simulink model "Simulink_StateDerivVec"  (R2022a)
settings: Solver=FixedStepAuto  StartTime=0.0  StopTime=timeEnd  FixedStep=SampleTime  RelTol=1e-6
values from neighbouring files (symbols this model uses):
  HorDistData = HorDistVec    [MainScript.m]    (also in MainScript_function.m)
  HorForceData = HorForceVec    [MainScript.m]    (also in MainScript_function.m)
  InitAIFactorVec = 1/3*ones(Farm.NumTurb,1)    [MainScript.m]    (also in MainScript_function.m)
  InitBladePitch = 0*ones(Farm.NumTurb,1)    [MainScript.m]    (also in MainScript_function.m)
  InitFreeStreamWindVel = Global.MeanWindSpeed    [MainScript.m]    (also in MainScript_function.m)
  InitGeneTorqueVec = 30000.*ones(Farm.NumTurb,1) * 97    [MainScript.m]    (also in MainScript_function.m)
  InitRotorSpeedVec = 1*ones(Farm.NumTurb,1)    [MainScript.m]    (also in MainScript_function.m)
  InitStateVec = [ ... (first row only)    [MainScript.m]    (also in MainScript_function.m)
  InitYawAngleVec = [-15;15;0]*pi/180    [MainScript.m]    (also in MainScript_function.m)
  modelselect = 1    [MainScript.m]    (also in MainScript_function.m)
  SampleTime = 1    [MainScript.m]    (also in MainScript_function.m)
settings Model: Creator=alich  LastModifiedBy=mluser
settings SolverCC: AlgebraicLoopSolver=LineSearch
settings DataIOCC: ExternalInput=Moor
settings DebuggingCC: UnconnectedInputMsg=warning  UnconnectedOutputMsg=warning  UnconnectedLineMsg=warning  SFMachineParentedDataDiag=warning
settings SFSimCC: CustomCodeUndefinedFunction=UseInterfaceOnly  DefaultCustomCodeDeterministicFunctions=All
settings RTWCC: GenCodeOnly=on  DLArmComputeVersion=19.05

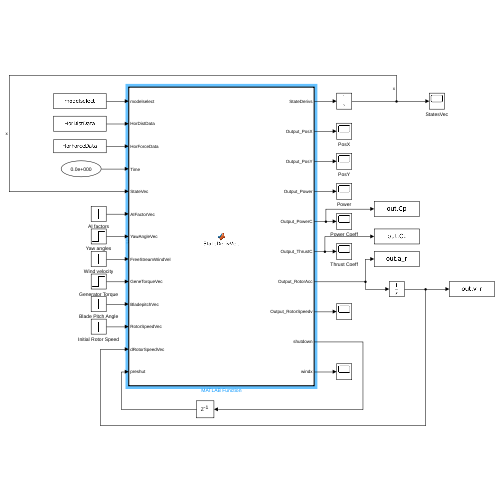
[thumbnail: Simulink's stored preview of the top-level diagram]
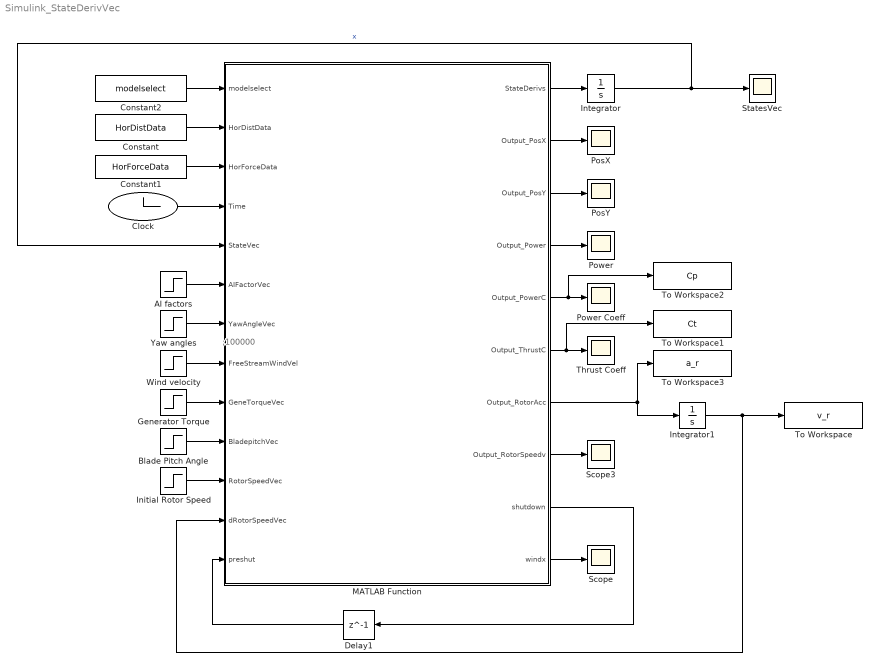
== system Simulink_StateDerivVec ==
  note: ;100000
  AI factors : Step  Time=0  Before=InitAIFactorVec  After=InitAIFactorVec  SampleTime=SampleTime
  Blade Pitch Angle : Step  Time=0  Before=InitBladePitch  After=InitBladePitch  SampleTime=SampleTime
  Clock : Clock
  Constant : Constant  Value=HorDistData  VectorParams1D=off
  Constant1 : Constant  Value=HorForceData  VectorParams1D=off
  Constant2 : Constant  Value=modelselect  SampleTime=SampleTime
  Delay1 : Delay  DelayLength=1  InitialCondition=0  SampleTime=SampleTime
  Generator Torque : Step  Time=0  Before=InitGeneTorqueVec  After=InitGeneTorqueVec  SampleTime=SampleTime
  Initial Rotor Speed : Step  Time=0  Before=InitRotorSpeedVec  After=InitRotorSpeedVec  SampleTime=SampleTime
  Integrator : Integrator  InitialCondition=InitStateVec  UpperSaturationLimit=100000  LowerSaturationLimit=0  IgnoreLimit=on
  Integrator1 : Integrator
  MATLAB Function : MATLAB Function  TreatAsAtomicUnit=on
  PosX : Scope
  PosY : Scope
  Power : Scope
  Power Coeff : Scope
  Scope : Scope
  Scope3 : Scope
  StatesVec : Scope
  Thrust Coeff : Scope
  To Workspace : ToWorkspace  VariableName=v_r  SaveFormat=Timeseries  SampleTime=-1
  To Workspace1 : ToWorkspace  VariableName=Ct  SaveFormat=Timeseries  SampleTime=-1
  To Workspace2 : ToWorkspace  VariableName=Cp  SaveFormat=Timeseries  SampleTime=-1
  To Workspace3 : ToWorkspace  VariableName=a_r  SaveFormat=Timeseries  SampleTime=-1
  Wind velocity : Step  Time=0  Before=[InitFreeStreamWindVel,0]  After=[InitFreeStreamWindVel,0]  SampleTime=SampleTime
  Yaw angles : Step  Time=0  Before=InitYawAngleVec  After=InitYawAngleVec  SampleTime=SampleTime
  wires:
  Clock/1 -> MATLAB Function/4(Time)
  MATLAB Function/1(StateDerivs) -> Integrator/1
  Integrator/1 -> MATLAB Function/5(StateVec), StatesVec/1  "x"
  MATLAB Function/2(Output_PosX) -> PosX/1
  MATLAB Function/3(Output_PosY) -> PosY/1
  MATLAB Function/4(Output_Power) -> Power/1
  AI factors/1 -> MATLAB Function/6(AIFactorVec)
  Yaw angles/1 -> MATLAB Function/7(YawAngleVec)
  Wind velocity/1 -> MATLAB Function/8(FreeStreamWindVel)
  MATLAB Function/5(Output_PowerC) -> Power Coeff/1, To Workspace2/1
  MATLAB Function/7(Output_RotorAcc) -> To Workspace3/1, Integrator1/1
  Initial Rotor Speed/1 -> MATLAB Function/11(RotorSpeedVec)
  Generator Torque/1 -> MATLAB Function/9(GeneTorqueVec)
  Integrator1/1 -> MATLAB Function/12(dRotorSpeedVec), To Workspace/1
  MATLAB Function/6(Output_ThrustC) -> Thrust Coeff/1, To Workspace1/1
  Blade Pitch Angle/1 -> MATLAB Function/10(BladepitchVec)
  MATLAB Function/8(Output_RotorSpeedv) -> Scope3/1
  MATLAB Function/9(shutdown) -> Delay1/1
  Delay1/1 -> MATLAB Function/13(preshut)
  MATLAB Function/10(windx) -> Scope/1
  Constant/1 -> MATLAB Function/2(HorDistData)
  Constant1/1 -> MATLAB Function/3(HorForceData)
  Constant2/1 -> MATLAB Function/1(modelselect)

== matlab function Simulink_StateDerivVec/MATLAB Function ==
  data: modelselect input; HorDistData input; HorForceData input; Time input; StateDerivs output; StateVec input; AIFactorVec input; YawAngleVec input; FreeStreamWindVel input; GeneTorqueVec input; BladepitchVec input; Output_PosX output; Output_PosY output; Output_Power output; Output_PowerC output; Output_ThrustC output; RotorSpeedVec input; Output_RotorAcc output; dRotorSpeedVec input; Output_RotorSpeedv output; preshut input; shutdown output; windx output
function [StateDerivs,Output_PosX,Output_PosY,Output_Power,Output_PowerC,Output_ThrustC,Output_RotorAcc,Output_RotorSpeedv,shutdown,windx]    = StateDerivVec(modelselect,HorDistData,HorForceData,Time,StateVec,AIFactorVec,YawAngleVec,FreeStreamWindVel,GeneTorqueVec,BladepitchVec,RotorSpeedVec,dRotorSpeedVec,preshut)
%% Load structures

Pars = load('Parameters_Simu.mat');

Solver = Pars.Solver; 
Global = Pars.Global;
Farm = Pars.Farm;
Turb = Pars.Turb;
Moor = Pars.Moor;
Arrays = Pars.Arrays;
TurbPosStateDerivMat = Arrays.TurbPosStateDerivMat;
TurbVelStateDerivMat = Arrays.TurbVelStateDerivMat;
WakeStateDerivMat = Arrays.WakeStateDerivMat;
TurbPowerVec = Arrays.TurbPowerVec;
WakeLocalVel = Arrays.WakeLocalVel;
WakeLocalAccel = Arrays.WakeLocalAccel;
WakeLocalDiaROT = Arrays.WakeLocalDiaROT;
Output_PosX = Arrays.Output_PosX;
Output_PosY = Arrays.Output_PosY;
Output_Power = Arrays.Output_Power;
Output_ThrustC=Arrays.Output_Power;
Output_PowerC=Arrays.Output_Power;
Output_RotorAcc=Arrays.Output_Power;
Output_RotorSpeedv = Arrays.Output_Power;
shutdown = Arrays.Output_Power;
windx = Arrays.Output_Power;

%if(modelselect==1)
data=load('paraVal.mat');
Lambda.mesh=data.paraVal.aero.lambda_grid;
Beta.mesh=data.paraVal.aero.beta_grid;
Cp.mesh=data.paraVal.aero.cp_grid;
Ct.mesh=data.paraVal.aero.ct_grid;
%end
   
%% Extract states and inputs
TurbPosMat = reshape(StateVec(1:2*Farm.NumTurb),2,Farm.NumTurb);
TurbVelMat = reshape(StateVec(2*Farm.NumTurb + 1:4*Farm.NumTurb),2,Farm.NumTurb);
WakeStateMat = reshape(StateVec(4*Farm.NumTurb + 1:4*Farm.NumTurb + 4*Farm.TotalNumWakePoints),4,Farm.TotalNumWakePoints);
for TurbNum = 1:Farm.NumTurb
 % Turbine states
 Turb(TurbNum).PosVec = TurbPosMat(:,TurbNum);
 Turb(TurbNum).VelVec = TurbVelMat(:,TurbNum);
 
 % Wake states
 Turb(TurbNum).WakePointPos_Y(1:Turb(TurbNum).NumWakePoints) = WakeStateMat(1,1:Turb(TurbNum).NumWakePoints);
 Turb(TurbNum).WakePointVelVec(:,1:Turb(TurbNum).NumWakePoints) = WakeStateMat(2:3,1:Turb(TurbNum).NumWakePoints);
 Turb(TurbNum).WakePointDia(1:Turb(TurbNum).NumWakePoints) = WakeStateMat(4,1:Turb(TurbNum).NumWakePoints);
 WakeStateMat(:,1:Turb(TurbNum).NumWakePoints) = [];
 
 % Turbine inputs
 Turb(TurbNum).YawAngle = YawAngleVec(TurbNum); %Yaw angle input is the same for both version of the model
 
 if(modelselect ==1) %3input
 Turb(TurbNum).BladePitch=BladepitchVec(TurbNum);
 Turb(TurbNum).GeneTorque=GeneTorqueVec(TurbNum);

 if (Time==0)
     Turb(TurbNum).RotorSpeed=RotorSpeedVec(TurbNum);
 else
     Turb(TurbNum).RotorSpeed=RotorSpeedVec(TurbNum)+dRotorSpeedVec(TurbNum);
     
 end
 else
     Turb(TurbNum).AIFactor = AIFactorVec(TurbNum);
 end
 
 end
 
% Free stream wind condition
Global.FreeStreamWindVel = FreeStreamWindVel; 
Global.FreeStreamWindAccel = [0 0]';

%% Define free stream wind unit vector
Global.FreeStreamUnitVec = Global.FreeStreamWindVel/norm(Global.FreeStreamWindVel);

%% Begin loop for state derivatives
BaseNum = 0;
for TurbNum = 1:Farm.NumTurb

 %% Calculate turbine platform state-derivatives
 % Incident wind velocity
 if (TurbNum == 1)
  Turb(TurbNum).UpsWindVelVec = Global.FreeStreamWindVel;
 else
  EffVelDeficit = 0;
  for UpsTurbNum = 1:TurbNum - 1
      if(preshut(TurbNum-1)==1&& UpsTurbNum>1)
     UpsTurbNum1 = UpsTurbNum-1;%check
      else
          UpsTurbNum1 = UpsTurbNum;
      end
      
   TurbPosXRelUpsTurb = Turb(TurbNum).PosVec(1) - Turb(UpsTurbNum1).PosVec(1);
   if TurbPosXRelUpsTurb >= 0
    UpsWakePosXData = [0 Turb(UpsTurbNum1).WakePointPos_X(1:Turb(TurbNum).NumWakePoints)];
    UpsWakePosYData = [0 Turb(UpsTurbNum1).WakePointPos_Y(1:Turb(TurbNum).NumWakePoints)];
    UpsWakeVelXData = [Turb(UpsTurbNum1).InitWakeVelVec(1) Turb(UpsTurbNum1).WakePointVelVec(1,1:Turb(TurbNum).NumWakePoints)];
    UpsWakeVelYData = [Turb(UpsTurbNum1).InitWakeVelVec(2) Turb(UpsTurbNum1).WakePointVelVec(2,1:Turb(TurbNum).NumWakePoints)];
    UpsWakeDiaData = [Turb(UpsTurbNum1).RotorDia Turb(UpsTurbNum1).WakePointDia(1:Turb(TurbNum).NumWakePoints)];
    
    for index = 1:length(UpsWakeVelXData) %in case of special numerical issue.
    if(isnan(UpsWakeVelXData(index))||isinf(UpsWakeVelXData(index)))
        UpsWakeVelXData(index) = 0;
    end
    end
    
    for indexs = 1:length(UpsWakeVelYData)
    if(isnan(UpsWakeVelYData(indexs))||isinf(UpsWakeVelYData(indexs)))
        UpsWakeVelYData(indexs) = 0;
    end
    end
    
    
    UpsWakePosY = Turb(UpsTurbNum1).PosVec(2) + interp1(UpsWakePosXData,UpsWakePosYData,TurbPosXRelUpsTurb,'Spline');
    UpsWakeVelX = Turb(UpsTurbNum1).VelVec(1) + interp1(UpsWakePosXData,UpsWakeVelXData,TurbPosXRelUpsTurb,'Spline');
    UpsWakeVelY = Turb(UpsTurbNum1).VelVec(2) + interp1(UpsWakePosXData,UpsWakeVelYData,TurbPosXRelUpsTurb,'Spline');
    UpsWakeDia = interp1(UpsWakePosXData,UpsWakeDiaData,TurbPosXRelUpsTurb,'Spline');
    UpsWakeOffset = abs(UpsWakePosY - Turb(TurbNum).PosVec(2));
    if UpsWakeOffset >= Turb(TurbNum).RotorDia/2 + UpsWakeDia/2
     EffVelVec = Global.FreeStreamWindVel;
    else
     b = Turb(TurbNum).RotorDia*(Global.GaussStd_Slope*TurbPosXRelUpsTurb/Turb(TurbNum).RotorDia + Global.GaussStd_Inter);
     a_x = 0.5*(((UpsWakeDia/2)/b)^2)*([1 0]*Global.FreeStreamWindVel - UpsWakeVelX);
     a_y = 0.5*(((UpsWakeDia/2)/b)^2)*([0 1]*Global.FreeStreamWindVel - UpsWakeVelY);
     UpsWakeVelX_Gauss = @(r) [1 0]*Global.FreeStreamWindVel - a_x*exp(-(r.^2)/(2*(b^2)));
     UpsWakeVelY_Gauss = @(r) [0 1]*Global.FreeStreamWindVel - a_y*exp(-(r.^2)/(2*(b^2)));
     Func_x = @(r) r.*AngleOLFunc(UpsWakeOffset,r,Turb(TurbNum).RotorDia/2).*UpsWakeVelX_Gauss(r);
     Func_y = @(r) r.*AngleOLFunc(UpsWakeOffset,r,Turb(TurbNum).RotorDia/2).*UpsWakeVelY_Gauss(r);
     r_vec = linspace(max(UpsWakeOffset - Turb(UpsTurbNum1).RotorDia/2,0),UpsWakeOffset + Turb(TurbNum).RotorDia/2,10);
     EffVelVec = [
      trapz(r_vec,Func_x(r_vec))/Turb(TurbNum).RotorArea;
      trapz(r_vec,Func_y(r_vec))/Turb(TurbNum).RotorArea];
     
    end
    EffVelDeficit =...
     EffVelDeficit + (norm(Global.FreeStreamWindVel)...
     - dot(EffVelVec,Global.FreeStreamUnitVec))^2;
   end
  end
  Turb(TurbNum).UpsWindVelVec =...
   (norm(Global.FreeStreamWindVel)...
   - sqrt(EffVelDeficit))*Global.FreeStreamUnitVec;

if(Turb(TurbNum).UpsWindVelVec(1)<0)
    Turb(TurbNum).UpsWindVelVec(1) = 0;
end
if(Turb(TurbNum).UpsWindVelVec(2)<0)
    Turb(TurbNum).UpsWindVelVec(2) = 0;
end


    
 end

 
 %% Ali's model to find Power and Thrust coefficients
 % Aerodynamic thrust force
 Turb(TurbNum).RelUpsWindVelVec = Turb(TurbNum).UpsWindVelVec - Turb(TurbNum).VelVec;
 Turb(TurbNum).RelWindAngle = atan(Turb(TurbNum).RelUpsWindVelVec(2)/Turb(TurbNum).RelUpsWindVelVec(1));
 Turb(TurbNum).RelYawAngle = Turb(TurbNum).YawAngle - Turb(TurbNum).RelWindAngle; %

 if(modelselect == 1)
 Turb(TurbNum).NormalWindVel = norm(Turb(TurbNum).RelUpsWindVelVec)*cos(Turb(TurbNum).RelYawAngle);%82
 Turb(TurbNum).Lambda = Turb(TurbNum).RotorSpeed*Turb(TurbNum).RotorDia/2/Turb(TurbNum).NormalWindVel;

 Turb(TurbNum).PowerCoeff = interp2(Beta.mesh,Lambda.mesh,Cp.mesh,Turb(TurbNum).BladePitch,Turb(TurbNum).Lambda);
 Turb(TurbNum).ThrustCoeff = interp2(Beta.mesh,Lambda.mesh,Ct.mesh,Turb(TurbNum).BladePitch,Turb(TurbNum).Lambda); 

 Turb(TurbNum).TurbTorque = 0.5*Global.AirDensity*Turb(TurbNum).RotorArea*(Turb(TurbNum).NormalWindVel)^3*Turb(TurbNum).PowerCoeff/Turb(TurbNum).RotorSpeed;
 Output_RotorAcc(TurbNum) = (Turb(TurbNum).TurbTorque-Turb(TurbNum).GeneTorque)/Turb(TurbNum).MomentInertia;

 if(isinf( Output_RotorAcc(TurbNum))||isnan( Output_RotorAcc(TurbNum)))
      Output_RotorAcc(TurbNum)=0;
      
 end
 else
    if(Turb(TurbNum).UpsWindVelVec(1)<=3) %%check
      Turb(TurbNum).AIFactor = 0;
    else
     Turb(TurbNum).AIFactor = AIFactorVec(TurbNum);
    end
  if strcmp(Solver.ActDiscModel,'Momentum')
  Turb(TurbNum).ThrustCoeff = 4*Turb(TurbNum).AIFactor*(cos(Turb(TurbNum).RelYawAngle) - Turb(TurbNum).AIFactor);
  Turb(TurbNum).PowerCoeff = 4*Turb(TurbNum).AIFactor*((cos(Turb(TurbNum).RelYawAngle) - Turb(TurbNum).AIFactor)^2); %fsolve
 elseif strcmp(Solver.ActDiscModel,'Glauert')
  Turb(TurbNum).ThrustCoeff = 4*Turb(TurbNum).AIFactor*sqrt(1 - Turb(TurbNum).AIFactor*(2*cos(Turb(TurbNum).RelYawAngle) - Turb(TurbNum).AIFactor));
  Turb(TurbNum).PowerCoeff = 4*Turb(TurbNum).AIFactor*(cos(Turb(TurbNum).RelYawAngle) - Turb(TurbNum).AIFactor)*sqrt(1 - Turb(TurbNum).AIFactor*(2*cos(Turb(TurbNum).RelYawAngle) - Turb(TurbNum).AIFactor));
 elseif strcmp(Solver.ActDiscModel,'Vortex')
  DefAngle = (0.6*Turb(TurbNum).AIFactor + 1)*Turb(TurbNum).RelYawAngle;
  Turb(TurbNum).ThrustCoeff = 4*Turb(TurbNum).AIFactor*(cos(Turb(TurbNum).RelYawAngle) + tan(DefAngle/2)*sin(Turb(TurbNum).RelYawAngle) - Turb(TurbNum).AIFactor*((sec(DefAngle/2))^2));
  Turb(TurbNum).PowerCoeff = 4*Turb(TurbNum).AIFactor*(cos(Turb(TurbNum).RelYawAngle) - Turb(TurbNum).AIFactor)*(cos(Turb(TurbNum).RelYawAngle) + tan(DefAngle/2)*sin(Turb(TurbNum).RelYawAngle) - Turb(TurbNum).AIFactor*((sec(DefAngle/2))^2));
 else
  error('Selected actuator disc model does not exist...');
  end
 end
     
 Turb(TurbNum).RotorNormVec = [
  cos(Turb(TurbNum).YawAngle);
  sin(Turb(TurbNum).YawAngle)];
 Turb(TurbNum).ThrustForceVec =...
  0.5*Turb(TurbNum).ThrustCoeff*Global.AirDensity*Turb(TurbNum).RotorArea*...
  (norm(Turb(TurbNum).RelUpsWindVelVec)^2)*Turb(TurbNum).RotorNormVec;
 
 
 % Hydrodynamic drag force
 Turb(TurbNum).DragForceVec = -Turb(TurbNum).EffDragFactor*norm(Turb(TurbNum).VelVec)*Turb(TurbNum).VelVec;
 LinDampForceVec = -1000000*Turb(TurbNum).VelVec;
 
 % Mooring line restoring force
 FLPosRelAnch1 = Turb(TurbNum).PosVec + Turb(TurbNum).FL1PosRelG - Turb(TurbNum).Anch1PosVec;
 FLPosRelAnch2 = Turb(TurbNum).PosVec + Turb(TurbNum).FL2PosRelG - Turb(TurbNum).Anch2PosVec;
 FLPosRelAnch3 = Turb(TurbNum).PosVec + Turb(TurbNum).FL3PosRelG - Turb(TurbNum).Anch3PosVec;
 Line1HorDist = norm(FLPosRelAnch1);
 Line2HorDist = norm(FLPosRelAnch2);
 Line3HorDist = norm(FLPosRelAnch3);
 Line1HorForce = interp1(HorDistData,HorForceData,Line1HorDist,'Spline');
 Line2HorForce = interp1(HorDistData,HorForceData,Line2HorDist,'Spline');
 Line3HorForce = interp1(HorDistData,HorForceData,Line3HorDist,'Spline');
 MoorForce1 = -Line1HorForce*FLPosRelAnch1/Line1HorDist;
 MoorForce2 = -Line2HorForce*FLPosRelAnch2/Line2HorDist;
 MoorForce3 = -Line3HorForce*FLPosRelAnch3/Line3HorDist;
 Turb(TurbNum).MoorForceVec = MoorForce1 + MoorForce2 + MoorForce3;
 
 % Turbine acceleration
 Turb(TurbNum).ForceVec = Turb(TurbNum).ThrustForceVec + Turb(TurbNum).MoorForceVec + Turb(TurbNum).DragForceVec...
     + LinDampForceVec;
 Turb(TurbNum).AccelVec = Solver.TurbMotion*Turb(TurbNum).ForceVec/(Turb(TurbNum).Mass + Turb(TurbNum).AddedMass);
 
 % Turbine power calculation
 
 if(modelselect ==1)
  if(preshut(TurbNum)==0)
 Turb(TurbNum).Power = Turb(TurbNum).RotorSpeed*Turb(TurbNum).GeneTorque;
 
 
 TurbPowerVec(TurbNum) = Turb(TurbNum).Power;
  else
  TurbPowerVec(TurbNum) = 0;
  end
 else
     Turb(TurbNum).Power = 0.5*Turb(TurbNum).PowerCoeff*Global.AirDensity*Turb(TurbNum).RotorArea*(norm(Turb(TurbNum).RelUpsWindVelVec)^3) + 5*(TurbPosMat(1, TurbNum) - Turb(TurbNum).PosVec(1)) + 5*(TurbPosMat(2, TurbNum) - Turb(TurbNum).PosVec(2));
 TurbPowerVec(TurbNum) = Turb(TurbNum).Power;
 %% calculate power coeff with 5MW -> calculate AI
 Maxpower = 5/0.994; % maximum rated power is 5MW
 Turb(TurbNum).PowerCoeff = Maxpower/(0.5*Global.AirDensity*Turb(TurbNum).RotorArea*(norm(Turb(TurbNum).RelUpsWindVelVec)^3));
 if strcmp(Solver.ActDiscModel,'Momentum')
  Turb(TurbNum).PowerCoeff = 4*Turb(TurbNum).AIFactor*((cos(Turb(TurbNum).RelYawAngle) - Turb(TurbNum).AIFactor)^2); %fsolve
 elseif strcmp(Solver.ActDiscModel,'Glauert')
  Turb(TurbNum).ThrustCoeff = 4*Turb(TurbNum).AIFactor*sqrt(1 - Turb(TurbNum).AIFactor*(2*cos(Turb(TurbNum).RelYawAngle) - Turb(TurbNum).AIFactor));
  Turb(TurbNum).PowerCoeff = 4*Turb(TurbNum).AIFactor*(cos(Turb(TurbNum).RelYawAngle) - Turb(TurbNum).AIFactor)*sqrt(1 - Turb(TurbNum).AIFactor*(2*cos(Turb(TurbNum).RelYawAngle) - Turb(TurbNum).AIFactor));
 elseif strcmp(Solver.ActDiscModel,'Vortex')
  DefAngle = (0.6*Turb(TurbNum).AIFactor + 1)*Turb(TurbNum).RelYawAngle;
  Turb(TurbNum).ThrustCoeff = 4*Turb(TurbNum).AIFactor*(cos(Turb(TurbNum).RelYawAngle) + tan(DefAngle/2)*sin(Turb(TurbNum).RelYawAngle) - Turb(TurbNum).AIFactor*((sec(DefAngle/2))^2));
  Turb(TurbNum).PowerCoeff = 4*Turb(TurbNum).AIFactor*(cos(Turb(TurbNum).RelYawAngle) - Turb(TurbNum).AIFactor)*(cos(Turb(TurbNum).RelYawAngle) + tan(DefAngle/2)*sin(Turb(TurbNum).RelYawAngle) - Turb(TurbNum).AIFactor*((sec(DefAngle/2))^2));
 else
  error('Selected actuator disc model does not exist...');
 end
 end
  
 %% Calculate wake state derivatives
 % Boundary condition at turbine
 if strcmp(Solver.RotorMomModel,'Jimenez')
  InitWakeVelMag = norm(Turb(TurbNum).RelUpsWindVelVec)*sqrt(abs(1 - Turb(TurbNum).ThrustCoeff));
  InitWakeAngle = -((cos(Turb(TurbNum).RelYawAngle))^2)*sin(Turb(TurbNum).RelYawAngle)*Turb(TurbNum).ThrustCoeff/2;
  Turb(TurbNum).InitWakeVelVec = InitWakeVelMag*[
   cos(InitWakeAngle + Turb(TurbNum).RelWindAngle);
   sin(InitWakeAngle + Turb(TurbNum).RelWindAngle)];
 elseif strcmp(Solver.RotorMomModel,'Bastankhah')
  InitWakeVelMag = norm(Turb(TurbNum).RelUpsWindVelVec)*sqrt(1 - Turb(TurbNum).ThrustCoeff);
  InitWakeAngle = -0.3*Turb(TurbNum).RelYawAngle/cos(Turb(TurbNum).RelYawAngle)*(1 - sqrt(1 - Turb(TurbNum).ThrustCoeff*cos(Turb(TurbNum).RelYawAngle)));
  Turb(TurbNum).InitWakeVelVec = InitWakeVelMag*[
   cos(InitWakeAngle + Turb(TurbNum).RelWindAngle);
   sin(InitWakeAngle + Turb(TurbNum).RelWindAngle)];
 else
  error('Selected momentum model does not exist...');
 end

 
 % Wake propagation
 for PointNum = 1:Turb(TurbNum).NumWakePoints
  PropVel = [1 0]*Global.FreeStreamWindVel - Turb(TurbNum).VelVec(1);
  WakeRecovGrad = (1/(pi/4*Turb(TurbNum).WakePointDia(PointNum)^2))*(pi/2*Turb(TurbNum).WakePointDia(PointNum)*Global.WakeExpRate)*(Global.FreeStreamWindVel - (Turb(TurbNum).VelVec + Turb(TurbNum).WakePointVelVec(:,PointNum)));
  if PointNum == 1
   WakeLocalVel(PointNum) = Turb(TurbNum).WakePointVelVec(2,PointNum) - PropVel*(Turb(TurbNum).WakePointPos_Y(PointNum + Solver.CentralDiff))/Turb(TurbNum).WakePointPos_X(PointNum + Solver.CentralDiff);
   WakeLocalAccel(:,PointNum) = Global.FreeStreamWindAccel - Turb(TurbNum).AccelVec - PropVel*(Turb(TurbNum).WakePointVelVec(:,PointNum + Solver.CentralDiff) - Turb(TurbNum).InitWakeVelVec)/Turb(TurbNum).WakePointPos_X(PointNum + Solver.CentralDiff) + WakeRecovGrad;
   WakeLocalDiaROT(PointNum) = Global.WakeExpRate - PropVel*(Turb(TurbNum).WakePointDia(PointNum + Solver.CentralDiff) - Turb(TurbNum).RotorDia)/Turb(TurbNum).WakePointPos_X(PointNum + Solver.CentralDiff);
  elseif PointNum == Turb(TurbNum).NumWakePoints
   WakeLocalVel(PointNum) = Turb(TurbNum).WakePointVelVec(2,PointNum) - PropVel*(Turb(TurbNum).WakePointPos_Y(PointNum) - Turb(TurbNum).WakePointPos_Y(PointNum - 1))/(Turb(TurbNum).WakePointPos_X(PointNum) - Turb(TurbNum).WakePointPos_X(PointNum - 1));
   WakeLocalAccel(:,PointNum) = Global.FreeStreamWindAccel - Turb(TurbNum).AccelVec - PropVel*(Turb(TurbNum).WakePointVelVec(:,PointNum) - Turb(TurbNum).WakePointVelVec(:,PointNum - 1))/(Turb(TurbNum).WakePointPos_X(PointNum) - Turb(TurbNum).WakePointPos_X(PointNum - 1)) + WakeRecovGrad;
   WakeLocalDiaROT(PointNum) = Global.WakeExpRate - PropVel*(Turb(TurbNum).WakePointDia(PointNum) - Turb(TurbNum).WakePointDia(PointNum - 1))/(Turb(TurbNum).WakePointPos_X(PointNum) - Turb(TurbNum).WakePointPos_X(PointNum - 1));
  else
   WakeLocalVel(PointNum) = Turb(TurbNum).WakePointVelVec(2,PointNum) - PropVel*(Turb(TurbNum).WakePointPos_Y(PointNum + Solver.CentralDiff) - Turb(TurbNum).WakePointPos_Y(PointNum - 1))/(Turb(TurbNum).WakePointPos_X(PointNum + Solver.CentralDiff) - Turb(TurbNum).WakePointPos_X(PointNum - 1));
   WakeLocalAccel(:,PointNum) = Global.FreeStreamWindAccel - Turb(TurbNum).AccelVec - PropVel*(Turb(TurbNum).WakePointVelVec(:,PointNum + Solver.CentralDiff) - Turb(TurbNum).WakePointVelVec(:,PointNum - 1))/(Turb(TurbNum).WakePointPos_X(PointNum + Solver.CentralDiff) - Turb(TurbNum).WakePointPos_X(PointNum - 1)) + WakeRecovGrad;
   WakeLocalDiaROT(PointNum) = Global.WakeExpRate - PropVel*(Turb(TurbNum).WakePointDia(PointNum + Solver.CentralDiff) - Turb(TurbNum).WakePointDia(PointNum - 1))/(Turb(TurbNum).WakePointPos_X(PointNum + Solver.CentralDiff) - Turb(TurbNum).WakePointPos_X(PointNum - 1));
  end
 end 
 
 % Build state derivative matrices
 TurbPosStateDerivMat(:,TurbNum) = Turb(TurbNum).VelVec;
 TurbVelStateDerivMat(:,TurbNum) = Turb(TurbNum).AccelVec;
 WakeStateDerivMat(:,BaseNum + 1:BaseNum + Turb(TurbNum).NumWakePoints) = [
  WakeLocalVel(1:Turb(TurbNum).NumWakePoints);
  WakeLocalAccel(:,1:Turb(TurbNum).NumWakePoints);
  WakeLocalDiaROT(1:Turb(TurbNum).NumWakePoints)];
 BaseNum = BaseNum + Turb(TurbNum).NumWakePoints;
end

%% Build final state derivative vector
StateDerivs = [
 reshape(TurbPosStateDerivMat,[],1);
 reshape(TurbVelStateDerivMat,[],1);
 reshape(WakeStateDerivMat,[],1)];
for i = 1: length(StateDerivs)
    if (isnan(StateDerivs(i))||isinf(StateDerivs(i))) 
        StateDerivs(i) = 0;
    end    
end

%% Outputs
for TurbNum = 1:Farm.NumTurb

    Output_PosX(TurbNum) = Turb(TurbNum).PosVec(1);
    Output_PosY(TurbNum) = Turb(TurbNum).PosVec(2);
    Output_Power(TurbNum) = Turb(TurbNum).Power;
    Output_ThrustC(TurbNum)=Turb(TurbNum).ThrustCoeff;
    Output_PowerC(TurbNum)=Turb(TurbNum).PowerCoeff;
    Output_RotorSpeedv(TurbNum)=Turb(TurbNum).RotorSpeed;
    windx(TurbNum)=Turb(TurbNum).UpsWindVelVec(1);
        if(Turb(TurbNum).UpsWindVelVec(1)>=3)
        shutdown(TurbNum)=0;
        else
        shutdown(TurbNum)=1;
        Output_Power(TurbNum) =0;
        end
end
